simulink model "calling_test"  (R2021a)
settings: Solver=FixedStepAuto  StartTime=0.0  StopTime=inf  FixedStep=.001  RelTol=1e-3
model workspace (MAT data in the model file):
  SL_ROS_VariableLengthArrays_MaxSizes.CommonInfo.ArrayTruncateAction = 'EmitWarning'
  SL_ROS_VariableLengthArrays_MaxSizes.MsgTypeMap = containers.Map
  SL_ROS_VariableLengthArrays_MaxSizes.MsgTypeMap.serialization.keys = {'rbdl_server/RBDLInverseDynamicsRequest'}
  SL_ROS_VariableLengthArrays_MaxSizes.MsgTypeMap.serialization.values{1}(1).PropertyName = 'ModelName'
  SL_ROS_VariableLengthArrays_MaxSizes.MsgTypeMap.serialization.values{1}(1).DataType = 'uint8'
  SL_ROS_VariableLengthArrays_MaxSizes.MsgTypeMap.serialization.values{1}(1).MaxLength = 3
  SL_ROS_VariableLengthArrays_MaxSizes.MsgTypeMap.serialization.values{1}(2).PropertyName = 'Q'
  SL_ROS_VariableLengthArrays_MaxSizes.MsgTypeMap.serialization.values{1}(2).DataType = 'double'
  SL_ROS_VariableLengthArrays_MaxSizes.MsgTypeMap.serialization.values{1}(2).MaxLength = 7
  SL_ROS_VariableLengthArrays_MaxSizes.MsgTypeMap.serialization.values{1}(3).PropertyName = 'Qd'
  SL_ROS_VariableLengthArrays_MaxSizes.MsgTypeMap.serialization.values{1}(3).DataType = 'double'
  SL_ROS_VariableLengthArrays_MaxSizes.MsgTypeMap.serialization.values{1}(3).MaxLength = 7
  SL_ROS_VariableLengthArrays_MaxSizes.MsgTypeMap.serialization.values{1}(4).PropertyName = 'Qdd'
  SL_ROS_VariableLengthArrays_MaxSizes.MsgTypeMap.serialization.values{1}(4).DataType = 'double'
  SL_ROS_VariableLengthArrays_MaxSizes.MsgTypeMap.serialization.values{1}(4).MaxLength = 7
  SL_ROS_VariableLengthArrays_MaxSizes.MsgTypeMap.serialization.uniformity = 0
  SL_ROS_VariableLengthArrays_MaxSizes.MsgTypeMap.serialization.keyType = 'char'
  SL_ROS_VariableLengthArrays_MaxSizes.MsgTypeMap.serialization.valueType = 'any'
undefined symbols (not defined in the file or in its folder): A, B, Q, Qd, Qdd
libraries: robotlib x4
settings Model: SimulationMode=external  Creator=nathaniel  LastModifiedBy=nathaniel
settings OptimizationCC: EnhancedBackFolding=on  PassReuseOutputArgsAs=Individual arguments  ZeroExternalMemoryAtStartup=off  ZeroInternalMemoryAtStartup=off  MaxStackSize=64  OptimizeBlockOrder=speed  DifferentSizesBufferReuse=on  OptimizationCustomize=off  EfficientTunableParamExpr=on
settings DebuggingCC: ParameterTunabilityLossMsg=error
settings HardwareCC: ProdBitPerPointer=32  ProdBitPerSizeT=32  ProdBitPerPtrDiffT=32  ProdLargestAtomicFloat=None  ProdIntDivRoundTo=Undefined  ProdEndianess=Unspecified  ProdWordSize=32  ProdHWDeviceType=Generic->Unspecified (assume 32-bit Generic)  TargetBitPerLong=64  TargetBitPerPointer=64  TargetBitPerSizeT=64  TargetBitPerPtrDiffT=64  TargetLongLongMode=on  TargetIntDivRoundTo=Zero  TargetEndianess=LittleEndian  TargetWordSize=64  TargetHWDeviceType=MATLAB Host  ProdEqTarget=off
settings ModelReferenceCC: ModelDependencies=/home/nathaniel/catkin_ws/src/ambf_walker
settings SFSimCC: MATLABDynamicMemAlloc=off
settings RTWCC: SystemTargetFile=ert.tlc  HardwareBoard=Robot Operating System (ROS)  TLCOptions="-aInlineSetEventsForThisBaseRateFcn=TLC_FALSE -aSuppressMultiTaskScheduler=TLC_FALSE  -aRateBasedStepFcn=0"  TemplateMakefile=ert_default_tmf  GenerateReport=on  RTWUseSimCustomCode=on  Toolchain=Catkin  TargetLang=C++
settings CodeAppCC: ForceParamTrailComments=on  IgnoreCustomStorageClasses=off  OperatorAnnotations=on  SimulinkDataObjDesc=on  SFDataObjDesc=on  InsertBlockDesc=on

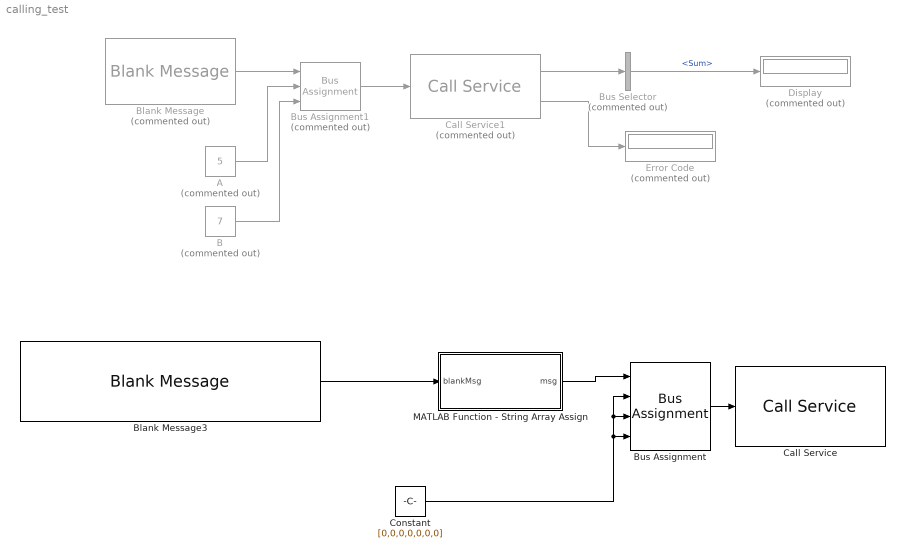
== system calling_test ==
  A : Constant  Commented=on  Value=5  OutDataTypeStr=double
  B : Constant  Commented=on  Value=7  OutDataTypeStr=double
  Blank Message : robotlib/Blank Message  Commented=on  messageClass=Service Request  entityType=ambf_walker/my_srv  messageType=ambf_walker/my_srvRequest  SampleTime=inf  legacyBusStruct=off
  Blank Message3 : robotlib/Blank Message  messageClass=Service Request  entityType=rbdl_server/RBDLInverseDynamics  messageType=rbdl_server/RBDLInverseDynamicsRequest  SampleTime=inf  legacyBusStruct=off
  Bus Assignment : BusAssignment  AssignedSignals=Q,Qd,Qdd
  Bus Assignment1 : BusAssignment  Commented=on  AssignedSignals=A,B
  Bus Selector : BusSelector  Commented=on  OutputSignals=Sum
  Call Service : robotlib/Call Service  topicSource=Specify your own  service=/my_service  serviceType=rbdl_server/RBDLInverseDynamics  connectionTimeout=5  keepPersistent=off  ShowErrorCodeOutput=on  legacyBusStruct=off
      settings: SourceProductBaseCode=RR
  Call Service1 : robotlib/Call Service  Commented=on  topicSource=Specify your own  service=/sum  serviceType=ambf_walker/my_srv  connectionTimeout=.001  keepPersistent=off  ShowErrorCodeOutput=on  legacyBusStruct=off
      settings: SourceProductBaseCode=RR
  Constant : Constant  Value=[0,0,0,0,0,0,0]
  Display : Display  Commented=on
  "Error Code " : Display  Commented=on
  MATLAB Function - String Array Assign : MATLAB Function  TreatAsAtomicUnit=on
  wires:
  Blank Message3/1 -> MATLAB Function - String Array Assign/1(blankMsg)
  MATLAB Function - String Array Assign/1(msg) -> Bus Assignment/1
  Constant/1 -> Bus Assignment/4, Bus Assignment/3, Bus Assignment/2
  Bus Assignment/1 -> Call Service/1
  B/1 -> Bus Assignment1/3
  Blank Message/1 -> Bus Assignment1/1
  Bus Assignment1/1 -> Call Service1/1
  Bus Selector/1 -> Display/1  "<Sum>"
  Call Service1/2 -> "Error Code "/1
  Call Service1/1 -> Bus Selector/1
  A/1 -> Bus Assignment1/2

== matlab function calling_test/MATLAB Function - String Array Assign ==
  data: blankMsg input; msg output Bus: SL_Bus_calling_test_rbdl_server_RBDLInverseDynamicsRequest
function msg = stringArrayAssign(blankMsg)
% stringArrayAssign - Assign a string array in a ROS message
%
%  blankMsg (input): A bus for a 'sensor_msgs/JointState' message. This is 
%      used to initialize the output.
%  msg (output): A bus for a 'sensor_msgs/JointState' message message, with 
%      Name field set to a string array.
%
%   Copyright 2015 The MathWorks, Inc.

%#codegen

% Note: The datatype of 'msg' has been explicitly set to the appropriate 
% Simulink bus type ("SL_Bus_robotROSMessageUsageExample_sensor_msgs_JointState"). 
%
% If the model name is changed, the datatype needs to be changed as well:
%   1) Click "Edit Data" in the Editor toolstrip to open "Ports and Data Manager"
%   2) Select "msg". From the "Type" dropdown, select "--- Refresh data types ---"
%   3) Set datatype to "Bus: SL_Bus_<modelname>_sensor_msgs_JointState"

strArrayToAssign = {'exo'};
msg = blankMsg;
name = 'exo';
strLength = length(name);
% Set the number of strings in the string array.
% msg (sensor_msgs/JointState) includes the following fields
%           Name : array of std_msgs/String (string array)
%   Name_SL_Info : struct with fields CurrentLength, ReceivedLength
numStringsInArray = length(strArrayToAssign);
msg.ModelName_SL_Info.CurrentLength = uint32(strLength); % uint32(numStringsInArray);

msg.ModelName(1:strLength) = uint8(name);
msg.Q_SL_Info.CurrentLength = uint32(7);
msg.Qd_SL_Info.CurrentLength = uint32(7);
msg.Qdd_SL_Info.CurrentLength = uint32(7);

% % Set the individual strings in the array
% for idx=1:numStringsInArray
%     str = strArrayToAssign{idx};
%     strLength = length(str);
%     msg.ModelName(idx).Data(1:strLength) = uint8(str);
%     msg.Name(idx).Data_SL_Info.CurrentLength = uint32(strLength);
% end
